simulink model "MultirotorSimPx4v1_8RateTuning"  (R2018b)
settings: Solver=VariableStepAuto  StartTime=0.0  StopTime=Simulation.T_END  MaxStep=Simulation.TS_MAX  RelTol=1e-3  EnableMultiTasking=on
PreLoadFcn:
  | % InitializeParameters;
undefined symbols (not defined in the file): Initial, Simulation, Uav
libraries: QuaternionLibrary x13, simulink_extras x10
(part 2 of 7)

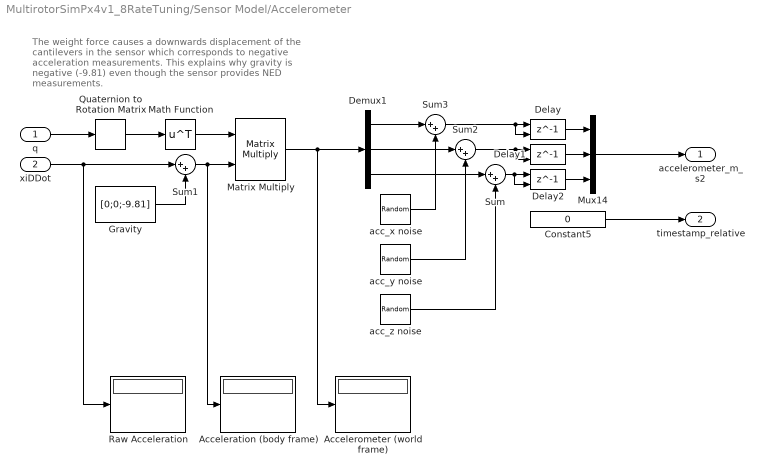
== system MultirotorSimPx4v1_8RateTuning/Sensor Model/Accelerometer ==
  note: The weight force causes a downwards displacement of
      | the cantilevers in the sensor which corresponds to
      | negative acceleration measurements. This explains why
      | gravity is negative (-9.81) even though the sensor provides
      | NED measurements.
  q : Inport
  xiDDot : Inport  Port=2  Unit=m/s^2
  Acceleration (body frame) : Display
  Accelerometer (world frame) : Display
  Constant5 : Constant  Value=0
  Delay : Delay  DelayLength=1  InitialConditionSource=Input port  SampleTime=1/400  StateName=accelerometerX
      settings: InputPortMap=u0,p4
  Delay1 : Delay  DelayLength=1  InitialConditionSource=Input port  SampleTime=1/400  StateName=accelerometerY
      settings: InputPortMap=u0,p4
  Delay2 : Delay  DelayLength=1  InitialConditionSource=Input port  SampleTime=1/400  StateName=accelerometerZ
      settings: InputPortMap=u0,p4
  Demux1 : Demux  Outputs=3
  Gravity : Constant  Value=[0;0;-9.81]
  Math Function : Math  Operator=transpose  SaturateOnIntegerOverflow=on
  Matrix Multiply : Product  Multiplication=Matrix(*)
  Mux14 : Mux  Inputs=3
  Quaternion to Rotation Matrix : QuaternionLibrary/Quaternion to Rotation Matrix
  Raw Acceleration : Display
  Sum{,1..3} (4 alike) : Sum  Inputs=|++
  acc_x noise : RandomNumber  Variance=0.012^2  SampleTime=1/400
  acc_y noise : RandomNumber  Variance=0.012^2  SampleTime=1/400
  acc_z noise : RandomNumber  Variance=0.02^2  SampleTime=1/400
  accelerometer_m_s2 : Outport  Unit=m/s^2  SampleTime=1/400
  timestamp_relative : Outport  Port=2  Unit=µs  SampleTime=1/400
  wires:
  Quaternion to Rotation Matrix/1 -> Math Function/1
  Math Function/1 -> Matrix Multiply/1
  Matrix Multiply/1 -> Demux1/1, Accelerometer (world frame)/1
  Gravity/1 -> Sum1/2
  Sum1/1 -> Acceleration (body frame)/1, Matrix Multiply/2
  Mux14/1 -> accelerometer_m_s2/1
  q/1 -> Quaternion to Rotation Matrix/1
  Constant5/1 -> timestamp_relative/1
  Demux1/1 -> Sum3/1
  Demux1/2 -> Sum2/1
  Demux1/3 -> Sum/1
  Sum/1 -> Delay2/2, Delay2/1
  acc_z noise/1 -> Sum/2
  Sum2/1 -> Delay1/2, Delay1/1
  Sum3/1 -> Delay/2, Delay/1
  acc_y noise/1 -> Sum2/2
  acc_x noise/1 -> Sum3/2
  Delay/1 -> Mux14/1
  Delay1/1 -> Mux14/2
  Delay2/1 -> Mux14/3
  xiDDot/1 -> Sum1/1, Raw Acceleration/1

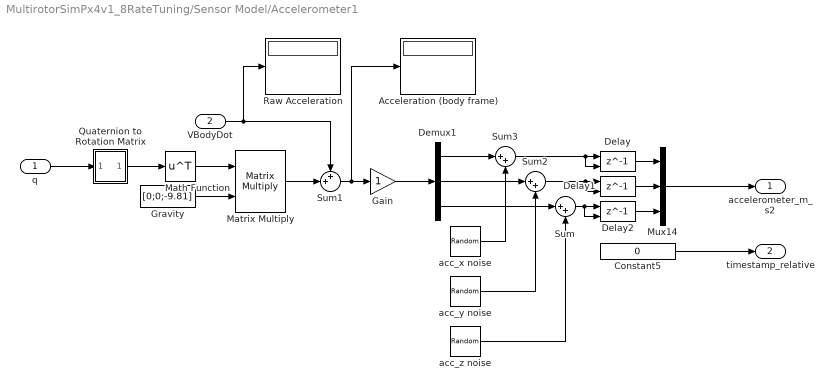
== system MultirotorSimPx4v1_8RateTuning/Sensor Model/Accelerometer1 ==
  q : Inport
  VBodyDot : Inport  Port=2  Unit=m/s^2
  Acceleration (body frame) : Display
  Constant5 : Constant  Value=0
  Delay : Delay  DelayLength=1  InitialConditionSource=Input port  SampleTime=1/400
      settings: InputPortMap=u0,p4
  Delay1 : Delay  DelayLength=1  InitialConditionSource=Input port  SampleTime=1/400
      settings: InputPortMap=u0,p4
  Delay2 : Delay  DelayLength=1  InitialConditionSource=Input port  SampleTime=1/400
      settings: InputPortMap=u0,p4
  Demux1 : Demux  Outputs=3
  Gain : Gain
  Gravity : Constant  Value=[0;0;-9.81]
  Math Function : Math  Operator=transpose  SaturateOnIntegerOverflow=on
  Matrix Multiply : Product  Multiplication=Matrix(*)
  Mux14 : Mux  Inputs=3
  Quaternion to Rotation Matrix : Subsystem  AncestorBlock=QuaternionLibrary/Quaternion to Rotation Matrix
      mask help: Convert an orientation quaternion to an orthogonal transformation matrix
      mask Help:
      | Convert an orientation quaternion
      | [q1 q2 q3 q4]
      | where:
      | - q1 is the rotation in radians
      | - [q2 q3 q4] is the vector around which the rotation is performed)
      | to an orthogonal transformation matrix
      | Based on code from the PX4 firmware: https://github.com/PX4/Firmware
      mask Display: disp('Q2R')
  Raw Acceleration : Display
  Sum : Sum  Inputs=|++
  Sum1 : Sum  Inputs=++|
  Sum2 : Sum  Inputs=|++
  Sum3 : Sum  Inputs=|++
  acc_x noise : RandomNumber  Variance=0.012^2  SampleTime=1/400
  acc_y noise : RandomNumber  Variance=0.012^2  SampleTime=1/400
  acc_z noise : RandomNumber  Variance=0.02^2  SampleTime=1/400
  accelerometer_m_s2 : Outport  Unit=m/s^2  SampleTime=1/400
  timestamp_relative : Outport  Port=2  Unit=µs  SampleTime=1/400
  wires:
  Quaternion to Rotation Matrix/1(rotationMatrix) -> Math Function/1
  Math Function/1 -> Matrix Multiply/1
  Matrix Multiply/1 -> Sum1/2
  Gravity/1 -> Matrix Multiply/2
  Mux14/1 -> accelerometer_m_s2/1
  q/1 -> Quaternion to Rotation Matrix/1(quaternion)
  Constant5/1 -> timestamp_relative/1
  Demux1/1 -> Sum3/1
  Demux1/2 -> Sum2/1
  Demux1/3 -> Sum/1
  Sum/1 -> Delay2/2, Delay2/1
  acc_z noise/1 -> Sum/2
  Sum2/1 -> Delay1/2, Delay1/1
  Sum3/1 -> Delay/2, Delay/1
  acc_y noise/1 -> Sum2/2
  acc_x noise/1 -> Sum3/2
  Delay/1 -> Mux14/1
  Delay1/1 -> Mux14/2
  Delay2/1 -> Mux14/3
  Sum1/1 -> Acceleration (body frame)/1, Gain/1
  VBodyDot/1 -> Raw Acceleration/1, Sum1/1
  Gain/1 -> Demux1/1

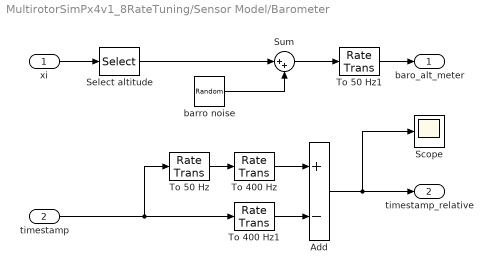
== system MultirotorSimPx4v1_8RateTuning/Sensor Model/Barometer ==
  xi : Inport  Unit=m
  timestamp : Inport  Port=2  Unit=µs
  Add : Sum  Inputs=+-
  Scope : Scope
  Select altitude : Selector  InputPortWidth=3  IndexOptions=Index vector (dialog)  Indices=3  OutputSizes=1
  Sum : Sum  Inputs=|++
  To 400 Hz : RateTransition  Deterministic=off  OutPortSampleTime=1/250
  To 400 Hz1 : RateTransition  OutPortSampleTime=1/400
  To 50 Hz : RateTransition  OutPortSampleTime=1/50
  To 50 Hz1 : RateTransition  OutPortSampleTime=1/50
  barro noise : RandomNumber  Variance=1/3^2  SampleTime=0.01
  baro_alt_meter : Outport  Unit=m  SampleTime=1/400
  timestamp_relative : Outport  Port=2  Unit=µs
  wires:
  barro noise/1 -> Sum/2
  Sum/1 -> To 50 Hz1/1
  xi/1 -> Select altitude/1
  Select altitude/1 -> Sum/1
  Add/1 -> timestamp_relative/1, Scope/1
  To 400 Hz1/1 -> Add/2
  To 50 Hz/1 -> To 400 Hz/1
  To 400 Hz/1 -> Add/1
  timestamp/1 -> To 50 Hz/1, To 400 Hz1/1
  To 50 Hz1/1 -> baro_alt_meter/1

== system MultirotorSimPx4v1_8RateTuning/Sensor Model/Global reprojection ==
  x : Inport
  y : Inport  Port=2
  map_projection_reproject : MATLAB Function  TreatAsAtomicUnit=on
  lat : Outport
  lon : Outport  Port=2
  wires:
  y/1 -> map_projection_reproject/2(y)
  map_projection_reproject/2(lon) -> lon/1
  x/1 -> map_projection_reproject/1(x)
  map_projection_reproject/1(lat) -> lat/1

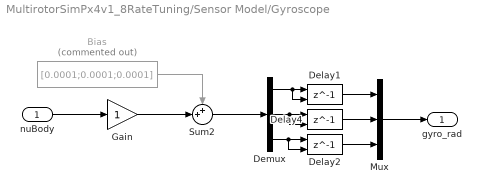
== system MultirotorSimPx4v1_8RateTuning/Sensor Model/Gyroscope ==
  nuBody : Inport  Unit=rad/s
  Bias : Constant  Commented=on  Value=[0.0001;0.0001;0.0001]
  Delay1 : Delay  DelayLength=1  InitialConditionSource=Input port  SampleTime=1/400  StateName=gyroX
      settings: InputPortMap=u0,p4
  Delay2 : Delay  DelayLength=1  InitialConditionSource=Input port  SampleTime=1/400  StateName=gyroZ
      settings: InputPortMap=u0,p4
  Delay4 : Delay  DelayLength=1  InitialConditionSource=Input port  SampleTime=1/400  StateName=gyroY
      settings: InputPortMap=u0,p4
  Demux : Demux  Outputs=3
  Gain : Gain
  Mux : Mux  Inputs=3
  Sum2 : Sum  Inputs=++|
  gyro_rad : Outport  Unit=rad/s  SampleTime=1/400
  wires:
  Sum2/1 -> Demux/1
  Mux/1 -> gyro_rad/1
  Bias/1 -> Sum2/1
  nuBody/1 -> Gain/1
  Delay4/1 -> Mux/2
  Delay2/1 -> Mux/3
  Delay1/1 -> Mux/1
  Demux/1 -> Delay1/2, Delay1/1
  Demux/2 -> Delay4/2, Delay4/1
  Demux/3 -> Delay2/2, Delay2/1
  Gain/1 -> Sum2/2

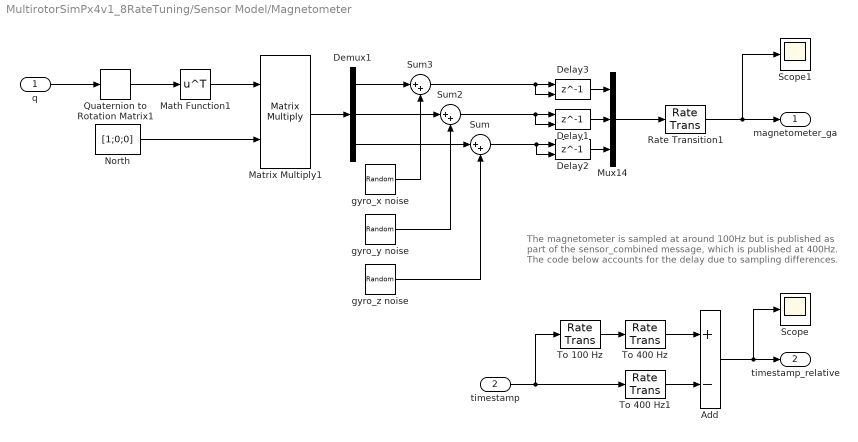
== system MultirotorSimPx4v1_8RateTuning/Sensor Model/Magnetometer ==
  note: The magnetometer is sampled at around 100Hz but is published
      | as part of the sensor_combined message, which is published at
      | 400Hz. The code below accounts for the delay due to sampling
      | differences.
  q : Inport
  timestamp : Inport  Port=2
  Add : Sum  Inputs=+-
  Delay1 : Delay  DelayLength=1  InitialConditionSource=Input port  SampleTime=1/100  StateName=magnetometerY
      settings: InputPortMap=u0,p4
  Delay2 : Delay  DelayLength=1  InitialConditionSource=Input port  SampleTime=1/100  StateName=magnetometerZ
      settings: InputPortMap=u0,p4
  Delay3 : Delay  DelayLength=1  InitialConditionSource=Input port  SampleTime=1/100  StateName=magnetometerX
      settings: InputPortMap=u0,p4
  Demux1 : Demux  Outputs=3
  Math Function1 : Math  Operator=transpose  SaturateOnIntegerOverflow=on
  Matrix Multiply1 : Product  Multiplication=Matrix(*)
  Mux14 : Mux  Inputs=3
  North : Constant  Value=[1;0;0]
  Quaternion to Rotation Matrix1 : QuaternionLibrary/Quaternion to Rotation Matrix
  Rate Transition1 : RateTransition  Deterministic=off  OutPortSampleTime=1/100
  Scope : Scope
  Scope1 : Scope
  Sum : Sum  Inputs=|++
  Sum2 : Sum  Inputs=|++
  Sum3 : Sum  Inputs=|++
  To 100 Hz : RateTransition  OutPortSampleTime=1/100
  To 400 Hz : RateTransition  Deterministic=off  OutPortSampleTime=1/250
  To 400 Hz1 : RateTransition  OutPortSampleTime=1/400
  gyro_x noise : RandomNumber  Variance=0.001^2  SampleTime=1/400
  gyro_y noise : RandomNumber  Variance=0.001^2  SampleTime=1/400
  gyro_z noise : RandomNumber  Variance=0.001^2  SampleTime=1/400
  magnetometer_ga : Outport  Unit=G  SampleTime=1/250
  timestamp_relative : Outport  Port=2  Unit=µs  SampleTime=1/250
  wires:
  q/1 -> Quaternion to Rotation Matrix1/1
  Quaternion to Rotation Matrix1/1 -> Math Function1/1
  North/1 -> Matrix Multiply1/2
  Math Function1/1 -> Matrix Multiply1/1
  Add/1 -> timestamp_relative/1, Scope/1
  Matrix Multiply1/1 -> Demux1/1
  Demux1/1 -> Sum3/1
  Demux1/2 -> Sum2/1
  Demux1/3 -> Sum/1
  Sum/1 -> Delay2/2, Delay2/1
  gyro_z noise/1 -> Sum/2
  Sum2/1 -> Delay1/2, Delay1/1
  gyro_y noise/1 -> Sum2/2
  gyro_x noise/1 -> Sum3/2
  Mux14/1 -> Rate Transition1/1
  To 400 Hz1/1 -> Add/2
  To 100 Hz/1 -> To 400 Hz/1
  To 400 Hz/1 -> Add/1
  Rate Transition1/1 -> Scope1/1, magnetometer_ga/1
  timestamp/1 -> To 100 Hz/1, To 400 Hz1/1
  Delay3/1 -> Mux14/1
  Sum3/1 -> Delay3/2, Delay3/1
  Delay1/1 -> Mux14/2
  Delay2/1 -> Mux14/3

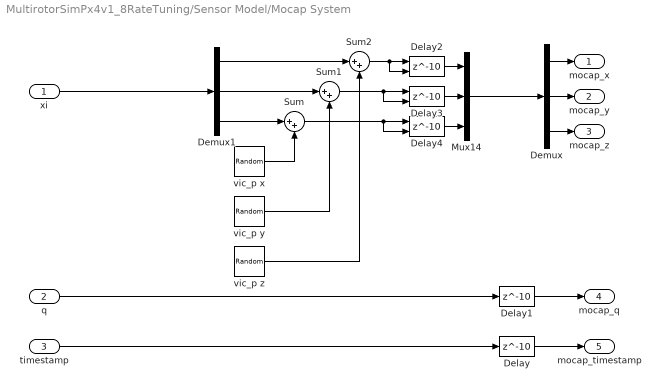
== system MultirotorSimPx4v1_8RateTuning/Sensor Model/Mocap System ==
  xi : Inport
  q : Inport  Port=2
  timestamp : Inport  Port=3
  Delay : Delay  DelayLength=10  SampleTime=1/100  StateName=mocapTimestamp
  Delay1 : Delay  DelayLength=10  SampleTime=1/100  StateName=mocapQ
  Delay2 : Delay  DelayLength=10  InitialConditionSource=Input port  SampleTime=1/100  StateName=mocapX
      settings: InputPortMap=u0,p4
  Delay3 : Delay  DelayLength=10  InitialConditionSource=Input port  SampleTime=1/100  StateName=mocapY
      settings: InputPortMap=u0,p4
  Delay4 : Delay  DelayLength=10  InitialConditionSource=Input port  SampleTime=1/100  StateName=mocapZ
      settings: InputPortMap=u0,p4
  Demux : Demux  Outputs=3
  Demux1 : Demux  Outputs=3
  Mux14 : Mux  Inputs=3
  Sum : Sum  Inputs=|++
  Sum1 : Sum  Inputs=|++
  Sum2 : Sum  Inputs=|++
  vic_p x : RandomNumber  Variance=0.001^2  SampleTime=0.01
  vic_p y : RandomNumber  Variance=0.001^2  SampleTime=0.01
  vic_p z : RandomNumber  Variance=0.001^2  SampleTime=0.01
  mocap_x : Outport
  mocap_y : Outport  Port=2
  mocap_z : Outport  Port=3
  mocap_q : Outport  Port=4
  mocap_timestamp : Outport  Port=5
  wires:
  q/1 -> Delay1/1
  timestamp/1 -> Delay/1
  Delay/1 -> mocap_timestamp/1
  Delay1/1 -> mocap_q/1
  Demux1/1 -> Sum2/1
  Demux1/2 -> Sum1/1
  xi/1 -> Demux1/1
  Demux1/3 -> Sum/1
  Sum/1 -> Delay4/2, Delay4/1
  vic_p x/1 -> Sum/2
  Sum1/1 -> Delay3/2, Delay3/1
  Sum2/1 -> Delay2/2, Delay2/1
  vic_p y/1 -> Sum1/2
  vic_p z/1 -> Sum2/2
  Demux/3 -> mocap_z/1
  Demux/2 -> mocap_y/1
  Demux/1 -> mocap_x/1
  Mux14/1 -> Demux/1
  Delay2/1 -> Mux14/1
  Delay3/1 -> Mux14/2
  Delay4/1 -> Mux14/3

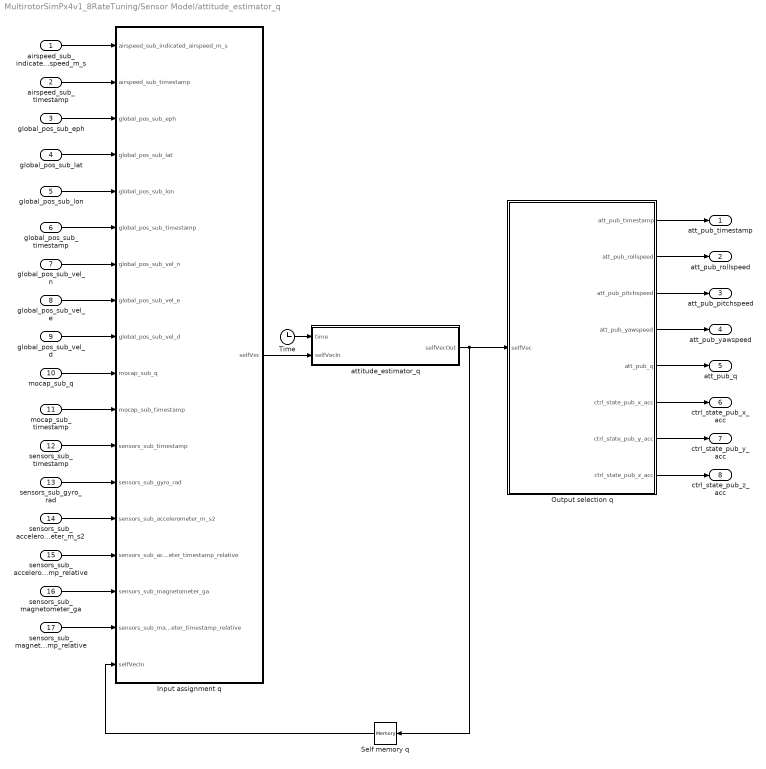
== system MultirotorSimPx4v1_8RateTuning/Sensor Model/attitude_estimator_q ==
  airspeed_sub_indicated_airspeed_m_s : Inport
  airspeed_sub_timestamp : Inport  Port=2
  global_pos_sub_eph : Inport  Port=3
  global_pos_sub_lat : Inport  Port=4
  global_pos_sub_lon : Inport  Port=5
  global_pos_sub_timestamp : Inport  Port=6
  global_pos_sub_vel_n : Inport  Port=7
  global_pos_sub_vel_e : Inport  Port=8
  global_pos_sub_vel_d : Inport  Port=9
  mocap_sub_q : Inport  Port=10
  mocap_sub_timestamp : Inport  Port=11
  sensors_sub_timestamp : Inport  Port=12
  sensors_sub_gyro_rad : Inport  Port=13
  sensors_sub_accelerometer_m_s2 : Inport  Port=14
  sensors_sub_accelerometer_timestamp_relative : Inport  Port=15
  sensors_sub_magnetometer_ga : Inport  Port=16
  sensors_sub_magnetometer_timestamp_relative : Inport  Port=17
  Input assignment q : MATLAB Function  TreatAsAtomicUnit=on
  Output selection q : MATLAB Function  TreatAsAtomicUnit=on
  Self memory q : Memory  InitialCondition=[ATT_ACC_COMP, 0, 0, 0, 0, 0, 0, 0, FW_ARSP_MODE, 0, 0, 0, 0, 0, 0, 0, 0, INIT_Q(1), INIT_Q(2), INIT_Q(3), INIT_Q(4), ATT_BIAS_MAX, 0, 0, INIT_Q(1), INIT_Q(2), INIT_Q(3), INIT_Q(4), 0, 0, 0, 0, 0, 0, 0, 0, 0, 0, 0, 0, 0.02, 0, ATT_EXT_HDG_M, 0, 0, 0, 0, 0, 0, 0, 0, 0, 0, 0, 0, 0, 0, 0, 0, 0, 0, 0, 0, 0, 0, 0, 0, 0, 0, 0, 0, 0, 0, 0, 0, 0, 0, 0, 0, 0, 0, 0, 0, 0, 0, 0, 0, 0, 0, 0, 0, 0, 0, 0, 0, 0, 0, 0, 0, 0, 0, 0, 0, 0, 0, 0, 0, 0, 0, 0, 0, 0, 0, 0, 0, 0, 0, 0, 0, 0, 0, 0, 0, 0, 0, 0, 0, 0, 0, 0, 0, 0, ATT_MAG_DECL, ATT_MAG_DECL_A, 0, 0, 0, 0, 0, 0, 0, 0, 0, 0, 0, 0, 0, 0, 0, 0, 0, 0, 0, 0, 0, 0, INIT_Q(1), INIT_Q(2), INIT_Q(3), INIT_Q(4), 0, 0, 0, 0, 0, 0, 0, 0, 0, 0, 0, 0, 0, 0, 0, 0, 0, 0, 0, 0, 0, 0, 0, 0, 0, 0, 0, 0, 0, 0, 0, 0, 0, 0, 0, 0, 0, 0, 0, ATT_W_ACC, ATT_W_EXT_HDG, ATT_W_GYRO_BIAS, ATT_W_MAG, 0, 0]
  Time : Clock
  attitude_estimator_q : MATLAB Function  TreatAsAtomicUnit=on  SystemSampleTime=Q_SAMPLING_PERIOD
  att_pub_timestamp : Outport
  att_pub_rollspeed : Outport  Port=2
  att_pub_pitchspeed : Outport  Port=3
  att_pub_yawspeed : Outport  Port=4
  att_pub_q : Outport  Port=5
  ctrl_state_pub_x_acc : Outport  Port=6
  ctrl_state_pub_y_acc : Outport  Port=7
  ctrl_state_pub_z_acc : Outport  Port=8
  wires:
  Output selection q/8(ctrl_state_pub_z_acc) -> ctrl_state_pub_z_acc/1
  Output selection q/7(ctrl_state_pub_y_acc) -> ctrl_state_pub_y_acc/1
  Output selection q/6(ctrl_state_pub_x_acc) -> ctrl_state_pub_x_acc/1
  Output selection q/5(att_pub_q) -> att_pub_q/1
  Output selection q/4(att_pub_yawspeed) -> att_pub_yawspeed/1
  Output selection q/3(att_pub_pitchspeed) -> att_pub_pitchspeed/1
  Output selection q/2(att_pub_rollspeed) -> att_pub_rollspeed/1
  Output selection q/1(att_pub_timestamp) -> att_pub_timestamp/1
  sensors_sub_magnetometer_timestamp_relative/1 -> Input assignment q/17(sensors_sub_magnetometer_timestamp_relative)
  sensors_sub_magnetometer_ga/1 -> Input assignment q/16(sensors_sub_magnetometer_ga)
  sensors_sub_accelerometer_timestamp_relative/1 -> Input assignment q/15(sensors_sub_accelerometer_timestamp_relative)
  sensors_sub_accelerometer_m_s2/1 -> Input assignment q/14(sensors_sub_accelerometer_m_s2)
  sensors_sub_gyro_rad/1 -> Input assignment q/13(sensors_sub_gyro_rad)
  sensors_sub_timestamp/1 -> Input assignment q/12(sensors_sub_timestamp)
  mocap_sub_timestamp/1 -> Input assignment q/11(mocap_sub_timestamp)
  mocap_sub_q/1 -> Input assignment q/10(mocap_sub_q)
  global_pos_sub_vel_d/1 -> Input assignment q/9(global_pos_sub_vel_d)
  global_pos_sub_vel_e/1 -> Input assignment q/8(global_pos_sub_vel_e)
  global_pos_sub_vel_n/1 -> Input assignment q/7(global_pos_sub_vel_n)
  global_pos_sub_timestamp/1 -> Input assignment q/6(global_pos_sub_timestamp)
  global_pos_sub_lon/1 -> Input assignment q/5(global_pos_sub_lon)
  global_pos_sub_lat/1 -> Input assignment q/4(global_pos_sub_lat)
  global_pos_sub_eph/1 -> Input assignment q/3(global_pos_sub_eph)
  airspeed_sub_timestamp/1 -> Input assignment q/2(airspeed_sub_timestamp)
  airspeed_sub_indicated_airspeed_m_s/1 -> Input assignment q/1(airspeed_sub_indicated_airspeed_m_s)
  Time/1 -> attitude_estimator_q/1(time)
  Self memory q/1 -> Input assignment q/18(selfVecIn)
  attitude_estimator_q/1(selfVecOut) -> Self memory q/1, Output selection q/1(selfVec)
  Input assignment q/1(selfVec) -> attitude_estimator_q/2(selfVecIn)

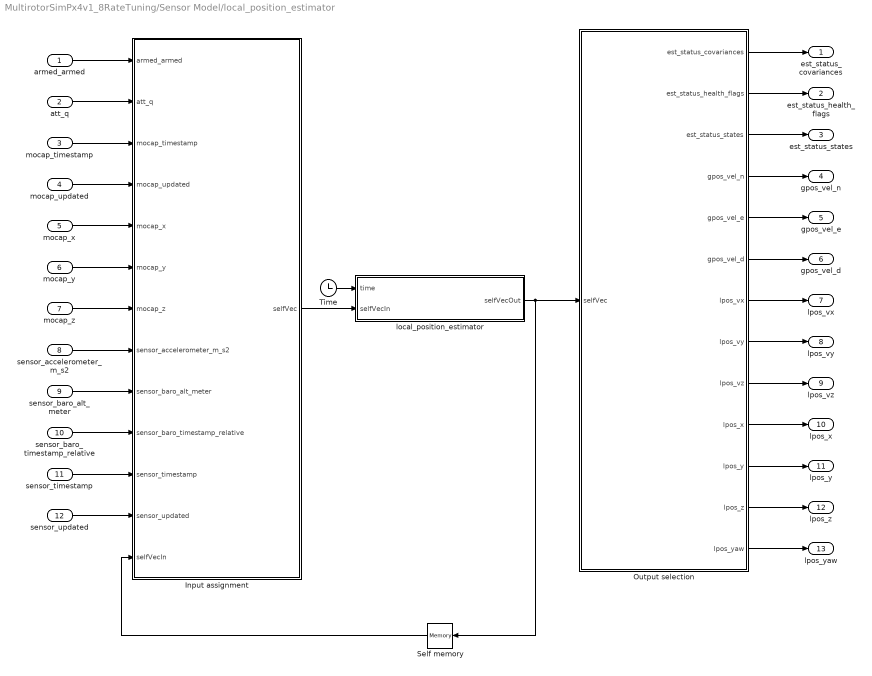
== system MultirotorSimPx4v1_8RateTuning/Sensor Model/local_position_estimator ==
  armed_armed : Inport
  att_q : Inport  Port=2
  mocap_timestamp : Inport  Port=3
  mocap_updated : Inport  Port=4
  mocap_x : Inport  Port=5
  mocap_y : Inport  Port=6
  mocap_z : Inport  Port=7
  sensor_accelerometer_m_s2 : Inport  Port=8
  sensor_baro_alt_meter : Inport  Port=9
  sensor_baro_timestamp_relative : Inport  Port=10
  sensor_timestamp : Inport  Port=11
  sensor_updated : Inport  Port=12
  Input assignment : MATLAB Function  TreatAsAtomicUnit=on
  Output selection : MATLAB Function  TreatAsAtomicUnit=on
  Self memory : Memory  InitialCondition=[0, 0, 0, 0, 0, 0, 0, 0, 0, 0, 0, 0, 0, 0, 0, 0, 0, 0, 0, 0, 0, 0, 0, 0, 0, 0, 0, 0, 0, 0, 0, 0, 0, 0, 0, 0, 0, 0, 0, 0, 0, 0, 0, 0, 0, 0, 0, 0, 0, 0, 0, 0, 0, 0, 0, 0, 0, 0, 0, 0, 0, 0, 0, 0, 0, 0, 0, 0, 0, 0, 0, 0, 0, 0, 0, 0, 0, 0, 0, 0, 0, 0, 0, 0, 0, 0, 0, 0, 0, 0, 0, 0, 0, 0, 0, 0, 0, 0, 0, 0, 0, 0, 0, 0, 0, 0, 0, 0, 0, 0, 0, 0, 0, 0, 0, 0, 0, 0, 0, 0, 0, 0, 0, 0, 0, 0, 0, 0, 0, 0, 0, 8.82050518214, 12.094592431, 13.9876612368, 16.0875642296, 17.8797700658, 19.6465647819, 1e-1, 2.0, 2.0, 2.0, 2^2, 2^0, 2^1, 2^7, 2^1, 2^6, 2^0, 2^4, 2^5, 2^2, 2^3, 0, 10.0, 8, 0, 0, 0, 0, 0, 0, 0, 0, 0, 0, 8, 0, 0, 0, 0, 0, 0, 0, 0, 0, 0, 8, 0, 0, 0, 0, 0, 0, 0, 0, 0, 0, 2*LPE_VXY_PUB*LPE_VXY_PUB, 0, 0, 0, 0, 0, 0, 0, 0, 0, 0, 2*LPE_VXY_PUB*LPE_VXY_PUB, 0, 0, 0, 0, 0, 0, 0, 0, 0, 0, 2*LPE_VXY_PUB*LPE_VXY_PUB, 0, 0, 0, 0, 0, 0, 0, 0, 0, 0, 1e-6, 0, 0, 0, 0, 0, 0, 0, 0, 0, 0, 1e-6, 0, 0, 0, 0, 0, 0, 0, 0, 0, 0, 1e-6, 0, 0, 0, 0, 0, 0, 0, 0, 0, 0, 8, 1.0e6, 0, 0, 0, 0, 0, 0, 0, 0, 0, 0, 0, 0, 0, 0, 0, 0, 0, 0, 0, 0, 0, 0, 0, 0, 0, 0, 0, 0, 0, 0, 0, 0, 0, 0, 0, 0, 0, 0, 0, 0, 0, 0, 0, 0, 0, 0, 0, 0, 0, 0, 0, 0, 0, 0, 0, 0, 0, 0, 0, 0, 0, 0, 0, 0, 0, 0, 0, 0, 0, 0, 0, 0, 0, 0, 0, 0, 0, 0, 0, 0, 0, 0, 0, 0, 0, 0, 0, 0, 0, 0, 0, 0, 0, 0, 0, 0, 0, 0, 0, 0, 0, 0, 0, 0, 0, 0, 0, 0, 0, 0, 0, 0, 0, 0, 0, 0, 0, 0, 2^0, 2^3, 2^1, 2^7, 2^2, 2^6, 2^4, 2^5, 0, LPE_ACC_XY, 0, LPE_ACC_Z, LPE_SAMPLING_PERIOD, LPE_X_LP, 0, 0, 0, 0, 0, 0, LPE_BAR_Z, LPE_SAMPLING_PERIOD, 0, 0, 0, 0, LPE_FAKE_ORIGIN, 0, LPE_FGYRO_HP, LPE_FGYRO_HP, LPE_FLW_QMIN, LPE_FLW_R, LPE_FLW_RR, LPE_FLW_SCALE, LPE_FLW_OFF_Z, LPE_FUSION, 0, LPE_GPS_DELAY, LPE_EPH_MAX, LPE_EPV_MAX, LPE_GPS_VXY, LPE_GPS_VZ, LPE_GPS_XY, LPE_GPS_Z, LPE_LAT, LPE_LON, 0, 0, LPE_LAND_VXY, LPE_LAND_Z, 0, LPE_LDR_OFF_Z, LPE_LDR_Z, 0, 0, 0, 0, 0, 0, 0, LPE_VIC_P, LPE_PN_B, LPE_PN_P, LPE_PN_T, LPE_PN_V, 8, 0, 0, 0, 0, 0, 0, 0, 0, 0, 0, 0, 0, 0, 0, 0, 0, 0, 0, 0, 0, 0, 0, 0, 0, 0, 0, 0, 0, 0, 0, 0, 0, 0, 0, 0, 0, 0, 0, 0, 0, 0, 0, 0, 0, 0, 0, 0, 0, 0, 0, 0, 0, 0, 0, 0, 0, 0, 0, 0, 0, 0, 0, 0, 0, 0, 0, 0, 0, 0, 0, 0, 0, 0, 0, 255, 0, LPE_SNR_OFF_Z, LPE_SNR_Z, 0, 0, 0, 0, 0, 0, 0, 0, 0, 0, 0, 0, 0, 0, 0, 0, 0, 0, 0, 0, 0, 0, 0, 0, 0, 0, 0, 0, 0, 0, 0, 0, 0, 0, 0, 0, 0, 0, 0, 1, 1, LPE_T_MAX_GRADE, 0, 0, 0, 0, 0, 0, 0, 0, 0, 0, 0, LPE_VIS_DELAY, LPE_VIS_XY, LPE_VIS_Z, LPE_VXY_PUB, 0, 0, 0, 0, 0, 0, 0, 0, 0, 0, 0, 0, 0, 0, 0, 0, 0, 0, 0, 0, 0, 0, 0, 0, 0, 0, 0, 0, 0, 0, 0, 0, 0, 0, 0, 0, 0, 0, 0, 0, 0, 0, 0, 0, 0, 0, 0, 0, 0, 0, 0, 0, 0, 0, 0, 0, 0, 0, 0, 0, 0, 0, 0, 0, 0, 0, 0, 0, 0, 0, 0, 0, 0, 0, 0, 0, 0, 0, 0, 0, 0, 0, 0, 0, 0, 0, 0, 0, 0, 0, 0, 0, 0, 0, 0, 0, 0, 0, 0, 0, 0, 0, 0, 0, 0, 0, 0, 0, 0, 0, 1, 1, LPE_SAMPLING_PERIOD, LPE_X_LP, 0, 0, 0, 0, 0, 0, 0, 0, 0, 0, LPE_Z_PUB]
  Time : Clock
  local_position_estimator : MATLAB Function  TreatAsAtomicUnit=on  SystemSampleTime=LPE_SAMPLING_PERIOD
  est_status_covariances : Outport
  est_status_health_flags : Outport  Port=2
  est_status_states : Outport  Port=3
  gpos_vel_n : Outport  Port=4
  gpos_vel_e : Outport  Port=5
  gpos_vel_d : Outport  Port=6
  lpos_vx : Outport  Port=7
  lpos_vy : Outport  Port=8
  lpos_vz : Outport  Port=9
  lpos_x : Outport  Port=10
  lpos_y : Outport  Port=11
  lpos_z : Outport  Port=12
  lpos_yaw : Outport  Port=13
  wires:
  Output selection/13(lpos_yaw) -> lpos_yaw/1
  Output selection/12(lpos_z) -> lpos_z/1
  Output selection/11(lpos_y) -> lpos_y/1
  Output selection/10(lpos_x) -> lpos_x/1
  Output selection/9(lpos_vz) -> lpos_vz/1
  Output selection/8(lpos_vy) -> lpos_vy/1
  Output selection/7(lpos_vx) -> lpos_vx/1
  Output selection/6(gpos_vel_d) -> gpos_vel_d/1
  Output selection/5(gpos_vel_e) -> gpos_vel_e/1
  Output selection/4(gpos_vel_n) -> gpos_vel_n/1
  Output selection/3(est_status_states) -> est_status_states/1
  Output selection/2(est_status_health_flags) -> est_status_health_flags/1
  Output selection/1(est_status_covariances) -> est_status_covariances/1
  sensor_updated/1 -> Input assignment/12(sensor_updated)
  sensor_timestamp/1 -> Input assignment/11(sensor_timestamp)
  sensor_baro_timestamp_relative/1 -> Input assignment/10(sensor_baro_timestamp_relative)
  sensor_baro_alt_meter/1 -> Input assignment/9(sensor_baro_alt_meter)
  sensor_accelerometer_m_s2/1 -> Input assignment/8(sensor_accelerometer_m_s2)
  mocap_z/1 -> Input assignment/7(mocap_z)
  mocap_y/1 -> Input assignment/6(mocap_y)
  mocap_x/1 -> Input assignment/5(mocap_x)
  mocap_updated/1 -> Input assignment/4(mocap_updated)
  mocap_timestamp/1 -> Input assignment/3(mocap_timestamp)
  att_q/1 -> Input assignment/2(att_q)
  armed_armed/1 -> Input assignment/1(armed_armed)
  Time/1 -> local_position_estimator/1(time)
  Self memory/1 -> Input assignment/13(selfVecIn)
  local_position_estimator/1(selfVecOut) -> Self memory/1, Output selection/1(selfVec)
  Input assignment/1(selfVec) -> local_position_estimator/2(selfVecIn)

== system MultirotorSimPx4v1_8RateTuning/Sensor Model/Accelerometer1/Quaternion to Rotation Matrix ==
  quaternion : Inport
  MATLAB Function : MATLAB Function  TreatAsAtomicUnit=on
  rotationMatrix : Outport
  wires:
  MATLAB Function/1(R) -> rotationMatrix/1
  quaternion/1 -> MATLAB Function/1(q)

== matlab function MultirotorSimPx4v1_8RateTuning/Quadrotor Quaternion Model/Equations of motion ==
  data: VBody input; VBodyDot output; nuBody input; Q input; TBody input size=3; tauBody input size=3; F_D input size=3; M_D input size=3; time input; nuBodyDot output; Uav parameter; xiDDot output; Simulation parameter
function [VBodyDot, nuBodyDot, xiDDot] = QuadrotorQuaternionModel(...
    VBody, nuBody, Q, TBody, tauBody, F_D, M_D, time, Uav, Simulation)
%#codegen

%% Handle 2D pitch test
if isfield( Uav, 'PITCH_ONLY') && Uav.PITCH_ONLY
    tauBody = [0; 1; 0] .* tauBody;
    M_D = [0; 1; 0] .* M_D;
end

if isfield( Simulation, 'T_START_STEP') && ( time < Simulation.T_START_STEP )
    tauBody = [0; 0; 0] .* tauBody;
    M_D = [0; 0; 0] .* M_D;
end

%% Moments and Forces
% Body frame accelerations
VBodyDot  = (1/Uav.M) * (Q'*Uav.G + TBody - cross(nuBody, Uav.M*VBody) + F_D);
nuBodyDot = Uav.I \ (tauBody - cross(nuBody, Uav.I*nuBody) + M_D);

% Inertial frame accelerations
xiDDot = (1/Uav.M)*(Uav.G + Q*(TBody + F_D));
% etaDDot = WInvertDot*nuBody + WInvert*nuBodyDot;

% Check centripetal force in inertial frame
% F_C = R*cross(nuBody,m*VBody);

if Uav.PITCH_ONLY
    xiDDot = [1; 1; 0] .* xiDDot;
end

end

== matlab function MultirotorSimPx4v1_8RateTuning/Compute Sph ==
  data: V_appBody input; azimuth output; elevation output; radius output
function [azimuth, elevation, radius] = computeSph(V_appBody)
%#codegen

% Convert from polar to spherical coordinates
[ azimuth, elevation, radius ] = cart2sph( V_appBody(1), V_appBody(2), V_appBody(3) );

== matlab function MultirotorSimPx4v1_8RateTuning/Applied wind speed/Relative velocity ==
  data: nuBody input; Uav parameter; VMotorRelBody output
function VMotorRelBody = relativeMotorVelocity( nuBody , Uav )
%#codegen
    VMotorRelBody = cross( nuBody, Uav.L_VEC );
end

== matlab function MultirotorSimPx4v1_8RateTuning/Applied wind speed/Compute V_app2 ==
  data: Q input; UBody output; U input size=3
function UBody = computeUBody(Q, U)
%#codegen

% Rotation matrix from Wind frame to Inertial frame
% Wind frame SEU, inertial frame NED
R_U = [1,  0, 0;
       0, -1, 0;
       0,  0, 1];
   
UBody = Q' * R_U * U;

== matlab function MultirotorSimPx4v1_8RateTuning/Sensor Model/Global reprojection/map_projection_reproject ==
  data: x input; y input; lat output; lon output; LAT0 parameter; LON0 parameter
function [ lat, lon ] = map_projection_reproject( x, y, LAT0, LON0)
%#codegen
%MAP_PROJECTION_REPROJECT
    M_DEG_TO_RAD = 0.017453292519943295;
	ref.lat_rad = LAT0 * M_DEG_TO_RAD;
	ref.lon_rad = LON0 * M_DEG_TO_RAD;
	ref.sin_lat = 0;
	ref.cos_lat = 0; 
    ref.sin_lat = sin(ref.lat_rad);
    ref.cos_lat = cos(ref.lat_rad);
    
    CONSTANTS_RADIUS_OF_EARTH = 6371000;
    M_PI = 3.14159265358979323846;

    x_rad = x / CONSTANTS_RADIUS_OF_EARTH;
    y_rad = y / CONSTANTS_RADIUS_OF_EARTH;
    c = sqrt(x_rad * x_rad + y_rad * y_rad);
    
    sin_c = sin(c);
    cos_c = cos(c);

    if (abs(c) > eps)
        lat_rad = asin(cos_c * ref.sin_lat + (x_rad * sin_c * ref.cos_lat) / c);
        lon_rad = (ref.lon_rad + atan2(y_rad * sin_c, c * ref.cos_lat * cos_c - x_rad * ref.sin_lat * sin_c));
    else
        lat_rad = ref.lat_rad;
        lon_rad = ref.lon_rad;
    end

    lat = lat_rad * 180.0 / M_PI;
    lon = lon_rad * 180.0 / M_PI;
end

== matlab function MultirotorSimPx4v1_8RateTuning/Sensor Model/attitude_estimator_q/Input assignment q ==
  data: airspeed_sub_indicated_airspeed_m_s input; airspeed_sub_timestamp input; global_pos_sub_eph input; global_pos_sub_lat input; global_pos_sub_lon input; global_pos_sub_timestamp input; global_pos_sub_vel_n input; global_pos_sub_vel_e input; global_pos_sub_vel_d input; mocap_sub_q input; mocap_sub_timestamp input; sensors_sub_timestamp input; sensors_sub_gyro_rad input; sensors_sub_accelerometer_m_s2 input; sensors_sub_accelerometer_timestamp_relative input; sensors_sub_magnetometer_ga input; sensors_sub_magnetometer_timestamp_relative input; selfVecIn input; selfVec output
function selfVec = InputAssignment( ...
	     airspeed_sub_indicated_airspeed_m_s, ...
	                  airspeed_sub_timestamp, ...
	                      global_pos_sub_eph, ...
	                      global_pos_sub_lat, ...
	                      global_pos_sub_lon, ...
	                global_pos_sub_timestamp, ...
	                    global_pos_sub_vel_n, ...
	                    global_pos_sub_vel_e, ...
	                    global_pos_sub_vel_d, ...
	                             mocap_sub_q, ...
	                     mocap_sub_timestamp, ...
	                   sensors_sub_timestamp, ...
	                    sensors_sub_gyro_rad, ...
	          sensors_sub_accelerometer_m_s2, ...
	sensors_sub_accelerometer_timestamp_relative, ...
	             sensors_sub_magnetometer_ga, ...
	sensors_sub_magnetometer_timestamp_relative, ...
	                               selfVecIn ...
	)
%#codegen

	selfVec = selfVecIn;

	% Variable assignment
	selfVec(10:10) =      airspeed_sub_indicated_airspeed_m_s;
	selfVec(11:11) =                   airspeed_sub_timestamp;
	selfVec(45:45) =                       global_pos_sub_eph;
	selfVec(46:46) =                       global_pos_sub_lat;
	selfVec(47:47) =                       global_pos_sub_lon;
	selfVec(48:48) =                 global_pos_sub_timestamp;
	selfVec(50:50) =                     global_pos_sub_vel_n;
	selfVec(51:51) =                     global_pos_sub_vel_e;
	selfVec(52:52) =                     global_pos_sub_vel_d;
	selfVec(147:150) =                              mocap_sub_q;
	selfVec(151:151) =                      mocap_sub_timestamp;
	selfVec(166:166) =                    sensors_sub_timestamp;
	selfVec(168:170) =                     sensors_sub_gyro_rad;
	selfVec(171:173) =           sensors_sub_accelerometer_m_s2;
	selfVec(174:174) = sensors_sub_accelerometer_timestamp_relative;
	selfVec(175:177) =              sensors_sub_magnetometer_ga;
	selfVec(178:178) = sensors_sub_magnetometer_timestamp_relative;
end

== matlab function MultirotorSimPx4v1_8RateTuning/Sensor Model/attitude_estimator_q/Output selection q ==
  data: att_pub_timestamp output; att_pub_rollspeed output; att_pub_pitchspeed output; att_pub_yawspeed output; att_pub_q output; selfVec input; ctrl_state_pub_x_acc output; ctrl_state_pub_y_acc output; ctrl_state_pub_z_acc output
function [ ...
                        att_pub_timestamp, ...
                        att_pub_rollspeed, ...
                       att_pub_pitchspeed, ...
                         att_pub_yawspeed, ...
                                att_pub_q, ...
                     ctrl_state_pub_x_acc, ...
                     ctrl_state_pub_y_acc, ...
                     ctrl_state_pub_z_acc] ...
   = OutputSelection( selfVec )
%#codegen

	% Variable assignment
	                       att_pub_timestamp = selfVec(14:14);
	                       att_pub_rollspeed = selfVec(15:15);
	                      att_pub_pitchspeed = selfVec(16:16);
	                        att_pub_yawspeed = selfVec(17:17);
	                               att_pub_q = selfVec(18:21);
	                    ctrl_state_pub_x_acc = selfVec(29:29);
	                    ctrl_state_pub_y_acc = selfVec(30:30);
	                    ctrl_state_pub_z_acc = selfVec(31:31);
end
